simulink model "SmartGridApplianceSimulationFallback"  (R2021a)
settings: Solver=ode45  StartTime=0  StopTime=5419320  RelTol=1e-3
settings Model: Creator=pankaja  LastModifiedBy=pankaja
settings DataIOCC: SaveFormat=StructureWithTime

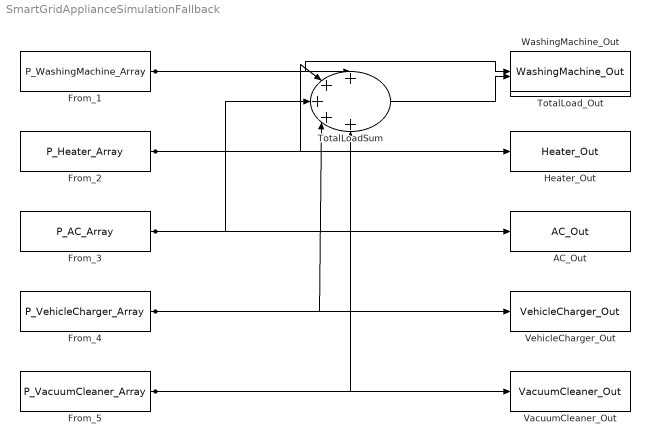
== system SmartGridApplianceSimulationFallback ==
  AC_Out : ToWorkspace  VariableName=AC_Out  SaveFormat=Structure With Time  SampleTime=-1
  From_1 : FromWorkspace  VariableName=P_WashingMachine_Array  SampleTime=-1
  From_2 : FromWorkspace  VariableName=P_Heater_Array  SampleTime=-1
  From_3 : FromWorkspace  VariableName=P_AC_Array  SampleTime=-1
  From_4 : FromWorkspace  VariableName=P_VehicleCharger_Array  SampleTime=-1
  From_5 : FromWorkspace  VariableName=P_VacuumCleaner_Array  SampleTime=-1
  Heater_Out : ToWorkspace  VariableName=Heater_Out  SaveFormat=Structure With Time  SampleTime=-1
  TotalLoadSum : Sum  Inputs=+++++
  TotalLoad_Out : ToWorkspace  VariableName=TotalLoad  SaveFormat=Structure With Time  SampleTime=-1
  VacuumCleaner_Out : ToWorkspace  VariableName=VacuumCleaner_Out  SaveFormat=Structure With Time  SampleTime=-1
  VehicleCharger_Out : ToWorkspace  VariableName=VehicleCharger_Out  SaveFormat=Structure With Time  SampleTime=-1
  WashingMachine_Out : ToWorkspace  VariableName=WashingMachine_Out  SaveFormat=Structure With Time  SampleTime=-1
  wires:
  From_1/1 -> WashingMachine_Out/1, TotalLoadSum/1
  From_2/1 -> Heater_Out/1, TotalLoadSum/2
  From_3/1 -> AC_Out/1, TotalLoadSum/3
  From_4/1 -> VehicleCharger_Out/1, TotalLoadSum/4
  From_5/1 -> VacuumCleaner_Out/1, TotalLoadSum/5
  TotalLoadSum/1 -> TotalLoad_Out/1
